simulink model "lane_keeping_fpga_in_the_loop"  (R2025b)
settings: Solver=ode1  StartTime=0.0  StopTime=30.0  RelTol=1e-3
model workspace (MAT data in the model file):
  firstWarning = 1
  originalScenarioChecksum = '9B63FD3C04BCEB1F00254244C35DE55B'
undefined symbols (not defined in the file): gray, Sim3dSensor
libraries: instrumentseriallib x3, simulink_extras x2, visiongeotforms x1, sim3dcameralib x1, sim3dlib x1, sim3dautolib x1
(part 1 of 2)
settings Model: Creator=aless  LastModifiedBy=corne

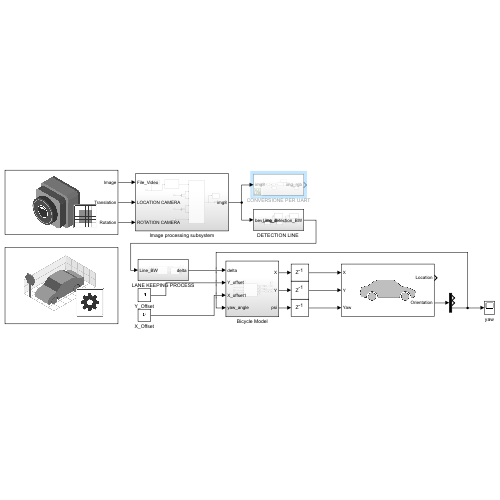
[thumbnail: Simulink's stored preview of the top-level diagram]
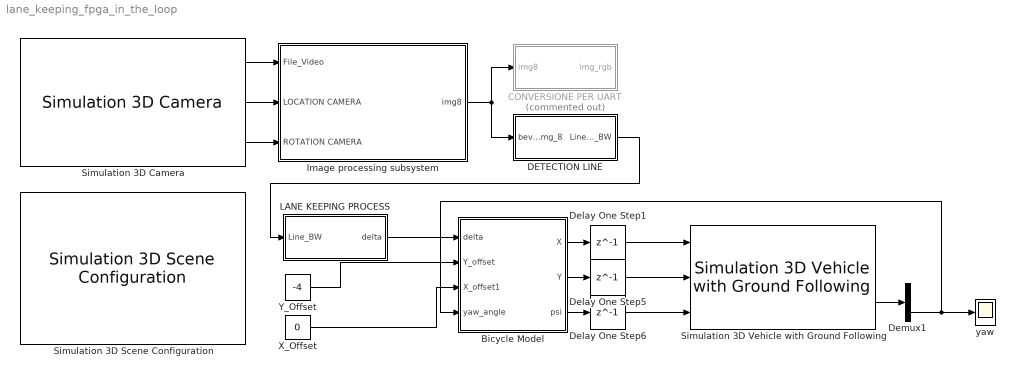
== system lane_keeping_fpga_in_the_loop ==
  Bicycle Model : Subsystem
  CONVERSIONE PER UART : Subsystem  Commented=on
  "DETECTION LINE " : Subsystem
  Delay One Step1 : Delay  DelayLength=1
  Delay One Step5 : Delay  DelayLength=1  InitialCondition=0
  Delay One Step6 : Delay  DelayLength=1
  Demux1 : Demux  Outputs=3
  Image processing subsystem : Subsystem
  LANE KEEPING PROCESS : Subsystem  Description=|
      | -Pulizia immagine
      | -Rotazione bev
      | -Pure pursuit
  Simulation 3D Camera : sim3dcameralib/Simulation 3D Camera  Priority=1  sensorTag=Sim3dSensor�  sensorId=1  sensorName=Sim3dSensor�  vehTagList={'Scene Origin';'ego'}  vehTag=ego  CoordinateSystem=ISO8855  mountLoc=Origin  offsetFlag=on  tmountOffset=[1.2,0,1.6]  extTmount=off  rmountOffset=[0.6,30,21.50]  extRmount=off  FocalLength=[950, 950]  OpticalCenter=[540, 960]  ImageSize=[1080, 1920]  RadialDistortion=[0, 0]  TangentialDistortion=[0, 0]  SensorSkew=0  VisualizeFieldOfView=off  FieldOfViewRange=61  DepthOutportEnabled=off  SemanticOutportEnabled=off  TransformOutportEnabled=on  SampleTime=-1  mountPoint=[1.2 0 1.6]  mountOrientation=[0.6 30 21.5]  aMode=3  ID=1
      settings: LibrarySourceBlock=drivingsim3d/Simulation 3D Camera
  Simulation 3D Scene Configuration : sim3dlib/Simulation 3D Scene Configuration  Priority=0  ProjectFormat=Default Scenes  SceneDesc=Straight road  ProjectName=C:\Program Files\MATLAB\R2025b\toolbox\shared\sim3d_projects\automotive_project_windows\UE\WindowsNoEditor\VehicleSimulation.exe  ScenePath=/Game/Maps/HwStrght  UEProjPath=C:\Users\aless\Desktop\AutoVrtlEnv\AutoVrtlEnv.uproject  EnableOpenDRIVE=off  OpenDRIVEName=C:\Users\aless\Desktop\acav\ACAV PROJECT\asam_prova\prova.xodr  vehTagList={'Custom';'Scene Origin';'ego'}  vehTag=ego  AttachedCameraRelativeTranslation=[0 0 0]  FreeCameraDefaultInitialTranslation=[-6, 0, 2]  AttachedCameraRelativeRotation=[0 0 0]  FreeCameraDefaultInitialRotation=[0, -15, 0]  ViewpointName=Custom  FreeCameraInitialTranslation=[0, 0, 0]  ViewpointTranslation=[0 0 0]  FreeCameraInitialRotation=[0, 0, 0]  ViewpointRotation=[0 0 0]  OpVisEn=off  Ts=1/100  EnableWindow=on  EnableRemoteAccess=off  EnableWeather=off  SunAzimuth=90  SunAltitude=40.0  EnableGeospatialSun=off  Latitude=0  Longitude=0  Date=2023-01-01  Time=10:30:00  GeoTimeZone=-5.0  SunDaylightSaving=off  wind=1  clouds=10  EnableVolumetricClouds=off  CloudCoverage=0  CloudAltitude=6  fog=0  rain=0  RaindropsEffect=off  SnowDensity=0  EnableGeospatial=off  TilesetSource=Earth terrain  UseTrueOrigin=off  OriginHeight=200  OriginLatitude=40.744652  OriginLongitude=-73.988864  MapStyle=Aerial  AdditionalAssetIDs=[]  UseAdvancedSunSky=off  SolarTime=11  TimeZone=-5  Day=21  Month=9  Year=2022  UseDaylightSavingTime=on  DSTStartDay=10  DSTStartMonth=3  DSTEndDay=3  DSTEndMonth=11  DSTSwitchHour=2  sensorTag=MainCamera1  sensorId=1  sensorName=MainCamera1  mountLoc=Origin  offsetFlag=off  tmountOffset=[0, 0, 0]  rmountOffset=[0, 0, 0]  HorizontalResolution=1280  VerticalResolution=720  HorizontalFOV=60  mountPoint=[0 0 0]  mountOrientation=[0 0 0]  aMode=3  ID=1  GeoTrigger=Inactive  ViewNameList={'Custom'}  ViewTranslationList={'[0 0 0]'}  ViewRotationList={'[0 0 0]'}
      settings: LibrarySourceBlock=drivingsim3d/Simulation 3D Scene Configuration
  Simulation 3D Vehicle with Ground Following : sim3dautolib/Simulation 3D Vehicle with Ground Following  Priority=-1  PassVehMesh=Sport utility vehicle  MeshPath=/MathWorksAutomotiveContent/Vehicles/Muscle/Meshes/SK_MuscleCar.SK_MuscleCar  TrackWidth=1.9  WheelBase=3  WheelRadius=0.35  VehColor=Red  CoordinateSystem=ISO8855  InitialPos=[0, -4, 0]  InitialRot=[0, 0, 0]  ActorName=ego  SampleTime=-1  ActorType=SimulinkVehicle  ID=C  aMode=3  ActorTag=ego  CoordinateScheme=0  VehLightsControl=off  HeadlightColor=[ 1, 1, 1 ]  HighBeamIntensity=100000  LowBeamIntensity=60000  HighBeamConeAngle=70  LowBeamConeAngle=70  LeftHeadlightOrientation=[ 0, 0 ]  RightHeadlightOrientation=[ 0, 0 ]  BrakelightIntensity=500  ReverselightIntensity=500  SignallightIntensity=500  SignallightPeriod=1  SignalPulseWidth=50  TransformOutportEnabled=on
      settings: LibrarySourceBlock=drivingsim3d/Simulation 3D Vehicle with Ground Following
  X_Offset : Constant  Value=0
  Y_Offset : Constant  Value=-4
  yaw : Scope
      settings: ActiveDisplayYMinimum=-1.1586010927242787  ActiveDisplayYMaximum=1.3448102951375731  DataLoggingVariableName=ScopeData11
  wires:
  "DETECTION LINE "/1(Line_detection_BW) -> LANE KEEPING PROCESS/1(Line_BW​)
  Image processing subsystem/1(img8) -> CONVERSIONE PER UART/1(img8), "DETECTION LINE "/1(bev_img_8)
  LANE KEEPING PROCESS/1(delta) -> Bicycle Model/1(delta)
  Simulation 3D Camera/1 -> Image processing subsystem/1(File_Video)
  Bicycle Model/2(Y) -> Delay One Step5/1
  Bicycle Model/1(X) -> Delay One Step1/1
  Simulation 3D Vehicle with Ground Following/2 -> Demux1/1
  Simulation 3D Camera/2 -> Image processing subsystem/2(LOCATION CAMERA)
  Simulation 3D Camera/3 -> Image processing subsystem/3(ROTATION CAMERA)
  Delay One Step6/1 -> Simulation 3D Vehicle with Ground Following/3
  Bicycle Model/3(psi) -> Delay One Step6/1
  Demux1/3 -> yaw/1, Bicycle Model/4(yaw_angle)
  Delay One Step1/1 -> Simulation 3D Vehicle with Ground Following/1
  Delay One Step5/1 -> Simulation 3D Vehicle with Ground Following/2
  Y_Offset/1 -> Bicycle Model/2(Y_offset)
  X_Offset/1 -> Bicycle Model/3(X_offset1)

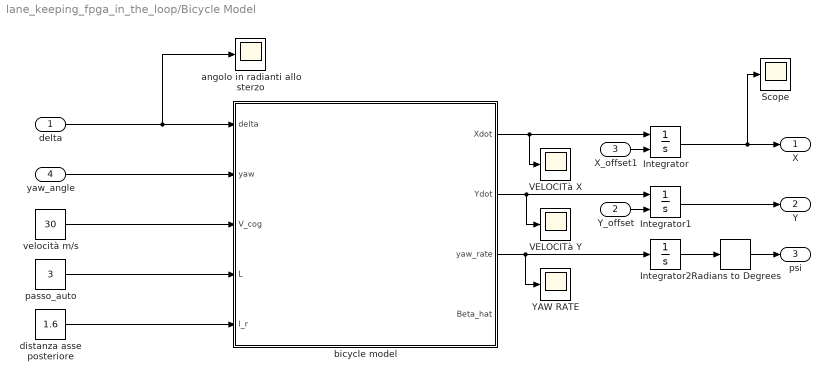
== system lane_keeping_fpga_in_the_loop/Bicycle Model ==
  delta : Inport
  Y_offset : Inport  Port=2
  X_offset1 : Inport  Port=3
  yaw_angle : Inport  Port=4
  Integrator : Integrator  InitialConditionSource=external
  Integrator1 : Integrator  InitialConditionSource=external  InitialCondition=-130
  Integrator2 : Integrator
  Radians to Degrees : simulink_extras/Transformations/Radians to Degrees
  Scope : Scope
      settings: ActiveDisplayYMinimum=-2.3618138795420052  ActiveDisplayYMaximum=7.426328435560519  DataLoggingVariableName=ScopeData5
  VELOCITà X : Scope
      settings: ActiveDisplayYMinimum=-0.055053619065674256  ActiveDisplayYMaximum=1.1172281798961861  DataLoggingVariableName=ScopeData3
  VELOCITà Y : Scope
      settings: ActiveDisplayYMinimum=-1  ActiveDisplayYMaximum=1  DataLoggingVariableName=ScopeData4
  YAW RATE : Scope
      settings: ActiveDisplayYMinimum=-0.13935375186428128  ActiveDisplayYMaximum=0.11342111745280879  DataLoggingVariableName=ScopeData2
  angolo in radianti allo sterzo : Scope
      settings: ActiveDisplayYMinimum=-0.34632467486503338  ActiveDisplayYMaximum=0.4914403733953655
  "bicycle model " : MATLAB Function  TreatAsAtomicUnit=on
  distanza asse posteriore : Constant  Value=1.6
  passo_auto : Constant  Value=3
  "velocità m/s " : Constant  Value=30
  X : Outport
  Y : Outport  Port=2
  psi : Outport  Port=3
  wires:
  "bicycle model "/1(Xdot) -> VELOCITà X/1, Integrator/1
  "bicycle model "/2(Ydot) -> VELOCITà Y/1, Integrator1/1
  Integrator/1 -> X/1, Scope/1
  Integrator1/1 -> Y/1
  delta/1 -> angolo in radianti allo sterzo/1, "bicycle model "/1(delta)
  yaw_angle/1 -> "bicycle model "/2(yaw)
  Radians to Degrees/1 -> psi/1
  "bicycle model "/3(yaw_rate) -> YAW RATE/1, Integrator2/1
  "velocità m/s "/1 -> "bicycle model "/3(V_cog)
  passo_auto/1 -> "bicycle model "/4(L)
  distanza asse posteriore/1 -> "bicycle model "/5(l_r)
  Integrator2/1 -> Radians to Degrees/1
  Y_offset/1 -> Integrator1/2
  X_offset1/1 -> Integrator/2

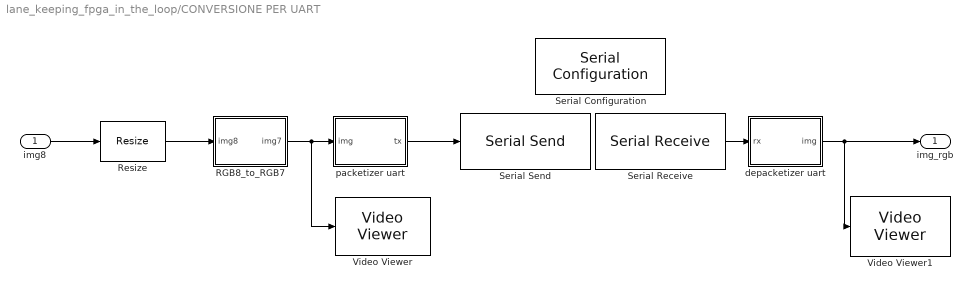
== system lane_keeping_fpga_in_the_loop/CONVERSIONE PER UART ==
  img8 : Inport
  RGB8_to_RGB7 : MATLAB Function  TreatAsAtomicUnit=on
  Resize : visiongeotforms/Resize  specify=Number of output rows and columns  rfactor=[200 150]  outCols=25  outRows=25  outRowsCols=[256 256]  interp_method=Bilinear  antialias=on  useROI=off  roiFlag=off  roundingMode=Nearest  overflowMode=on  prodOutputMode=Binary point scaling  prodOutputWordLength=32  prodOutputFracLength=10
  Serial Configuration : instrumentseriallib/Serial Configuration  Description=il valore del baund rate è uguale a fpga (la massima è 921600 e dipende da usb pc non da fpga)  Priority=-200000  PortSel=COM5  Port=COM5  ComPort=COM5  BaudRate=921600  DataBits=8  Parity=none  StopBits=1  ByteOrder=little-endian  FlowControl=none  Timeout=10  SimulateUsing=Interpreted execution  BlockInModel=on  aMode=1
  Serial Receive : instrumentseriallib/Serial Receive  Priority=1  PortSel=COM5  Port=COM5  ComPort=COM5  DataType=uint8  SaveDataType=uint8  ToggleHeader=on  Header=[255]  ToggleDataSize=on  DataSize=[65536 1]  ToggleTerminator=on  Terminator=Custom terminator  CustomTerminator=[241]  InputFormat=Column major  EnableBlockingMode=on  ActionDataUnavailable=Output last received value  ActionWhenDataUnavailable=Output last received value  CustomValue=0  SampleTime=0.1  SimulateUsing=Interpreted execution  BlockInModel=on  aMode=1  LibraryInUse=instrumentlib
  Serial Send : instrumentseriallib/Serial Send  Priority=1  PortSel=COM5  Port=COM5  ComPort=COM5  Header=[255]  Terminator=Custom terminator  CustomTerminator=[241]  EnableBlockingMode=off  SimulateUsing=Interpreted execution  BlockInModel=on  aMode=1
  Video Viewer : VideoViewer  Description=test di controllo RGB a 7 bit (da 8 bit eseguiamo una divisione per 2 perchè 1 bit degli 8 inviati indica che è l'ultimo bit inviato)  colormapValue=gray(256)  FigPos=[1019 931.666666666667 645 275]
  Video Viewer1 : VideoViewer  colormapValue=gray(256)  FigPos=[878 553.666666666667 845 301]
  depacketizer uart : MATLAB Function  TreatAsAtomicUnit=on
  packetizer uart : MATLAB Function  TreatAsAtomicUnit=on
  img_rgb : Outport
  wires:
  RGB8_to_RGB7/1(img7) -> packetizer uart/1(img), Video Viewer/1
  Serial Receive/1 -> depacketizer uart/1(rx)
  depacketizer uart/1(img) -> Video Viewer1/1, img_rgb/1
  Resize/1 -> RGB8_to_RGB7/1(img8)
  img8/1 -> Resize/1
  packetizer uart/1(tx) -> Serial Send/1

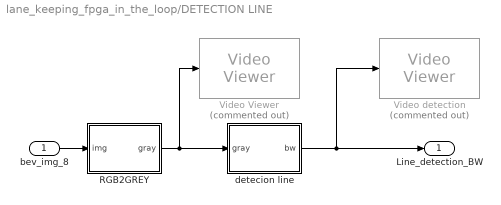
== system lane_keeping_fpga_in_the_loop/DETECTION LINE  ==
  bev_img_8 : Inport
  RGB2GREY : MATLAB Function  TreatAsAtomicUnit=on
  Video Viewer : VideoViewer  Commented=on  colormapValue=gray(256)  FigPos=[1270 462.666666666667 418 304]
  Video detection : VideoViewer  Commented=on  colormapValue=gray(256)  FigPos=[856 1015.66666666667 851 911]
  detecion line : MATLAB Function  TreatAsAtomicUnit=on
  Line_detection_BW : Outport
  wires:
  bev_img_8/1 -> RGB2GREY/1(img)
  RGB2GREY/1(gray) -> Video Viewer/1, detecion line/1(gray)
  detecion line/1(bw) -> Line_detection_BW/1, Video detection/1

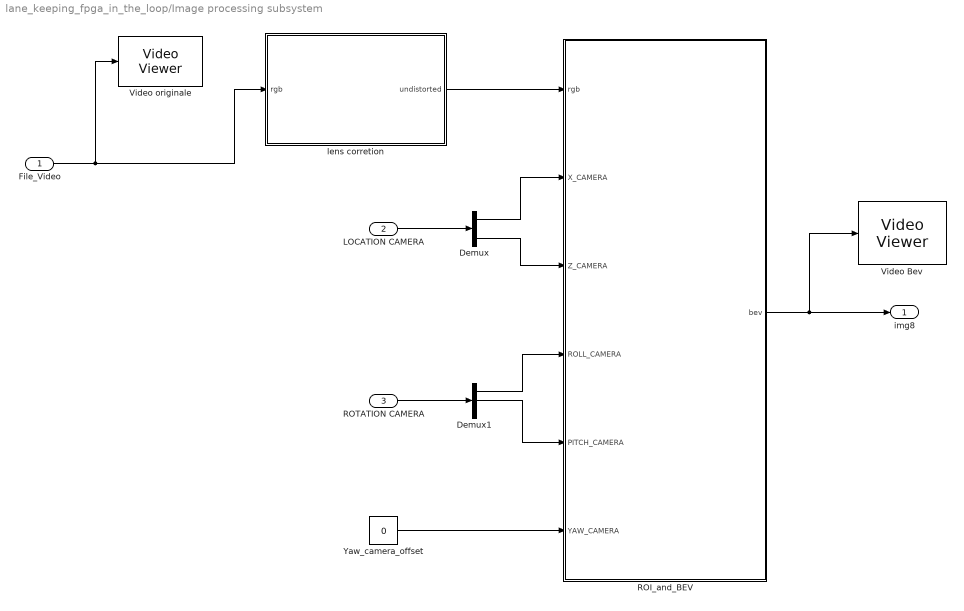
== system lane_keeping_fpga_in_the_loop/Image processing subsystem ==
  File_Video : Inport
  LOCATION CAMERA : Inport  Port=2
  ROTATION CAMERA : Inport  Port=3
  Demux : Demux  Outputs=3
  Demux1 : Demux  Outputs=3
  ROI_and_BEV : MATLAB Function  TreatAsAtomicUnit=on
  Video Bev : VideoViewer  colormapValue=gray(256)  FigPos=[-13 965 1539 768]
  Video originale : VideoViewer  colormapValue=gray(256)  FigPos=[1 814 1536 717]
  Yaw_camera_offset : Constant  Value=0
  lens corretion : MATLAB Function  TreatAsAtomicUnit=on
  img8 : Outport
  wires:
  File_Video/1 -> Video originale/1, lens corretion/1(rgb)
  LOCATION CAMERA/1 -> Demux/1
  lens corretion/1(undistorted) -> ROI_and_BEV/1(rgb)
  ROI_and_BEV/1(bev) -> img8/1, Video Bev/1
  Demux/1 -> ROI_and_BEV/2(X_CAMERA)
  Demux/3 -> ROI_and_BEV/3(Z_CAMERA)
  ROTATION CAMERA/1 -> Demux1/1
  Demux1/1 -> ROI_and_BEV/4(ROLL_CAMERA)
  Demux1/2 -> ROI_and_BEV/5(PITCH_CAMERA)
  Yaw_camera_offset/1 -> ROI_and_BEV/6(YAW_CAMERA)

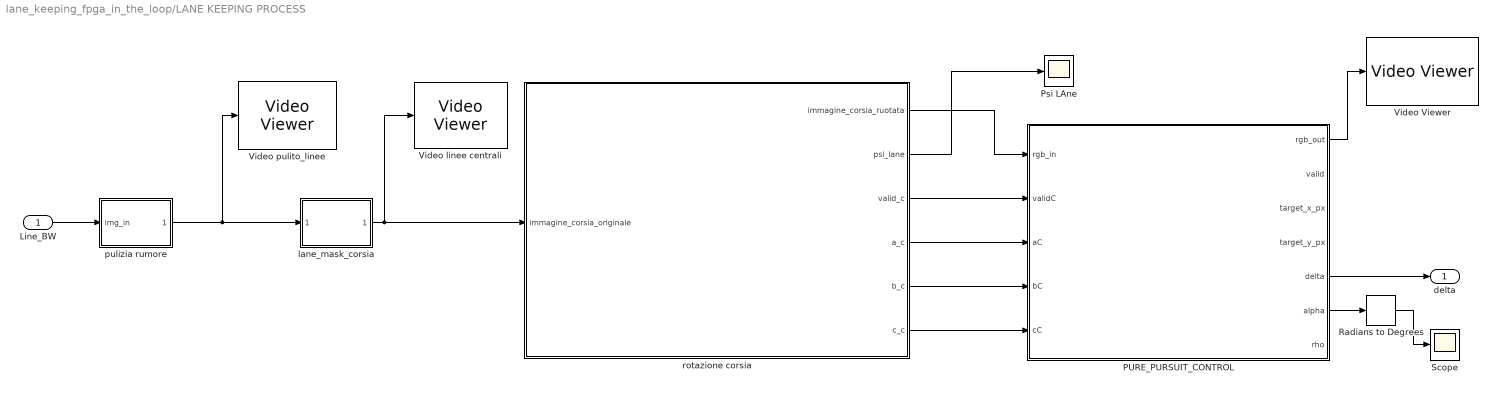
== system lane_keeping_fpga_in_the_loop/LANE KEEPING PROCESS ==
  Line_BW​ : Inport
  PURE_PURSUIT_CONTROL : MATLAB Function  TreatAsAtomicUnit=on
  Psi LAne : Scope
  Radians to Degrees : simulink_extras/Transformations/Radians to Degrees
  Scope : Scope
      settings: ActiveDisplayYMinimum=-21.688585463495443  ActiveDisplayYMaximum=29.571917697196469  DataLoggingVariableName=ScopeData8
  Video Viewer : VideoViewer  colormapValue=gray(256)  FigPos=[1024 631 383 351]
  Video linee centrali : VideoViewer  colormapValue=gray(256)  FigPos=[591 907 851 768]
  Video pulito_linee : VideoViewer  colormapValue=gray(256)  FigPos=[2 1015.66666666667 851 767.66666666667]
  lane_mask_corsia : MATLAB Function  TreatAsAtomicUnit=on
  pulizia rumore : MATLAB Function  TreatAsAtomicUnit=on
  rotazione corsia : Subsystem
  delta : Outport
  wires:
  Line_BW​/1 -> pulizia rumore/1(img_in)
  lane_mask_corsia/1(lane_mask) -> Video linee centrali/1, rotazione corsia/1(immagine_corsia_originale)
  rotazione corsia/1(immagine_corsia_ruotata) -> PURE_PURSUIT_CONTROL/1(rgb_in)
  rotazione corsia/2(psi_lane) -> Psi LAne/1
  rotazione corsia/3(valid_c) -> PURE_PURSUIT_CONTROL/2(validC)
  rotazione corsia/4(a_c) -> PURE_PURSUIT_CONTROL/3(aC)
  rotazione corsia/5(b_c) -> PURE_PURSUIT_CONTROL/4(bC)
  rotazione corsia/6(c_c) -> PURE_PURSUIT_CONTROL/5(cC)
  PURE_PURSUIT_CONTROL/1(rgb_out) -> Video Viewer/1
  Radians to Degrees/1 -> Scope/1
  PURE_PURSUIT_CONTROL/5(delta) -> delta/1
  PURE_PURSUIT_CONTROL/6(alpha) -> Radians to Degrees/1
  pulizia rumore/1(img_out) -> Video pulito_linee/1, lane_mask_corsia/1(binary_img)

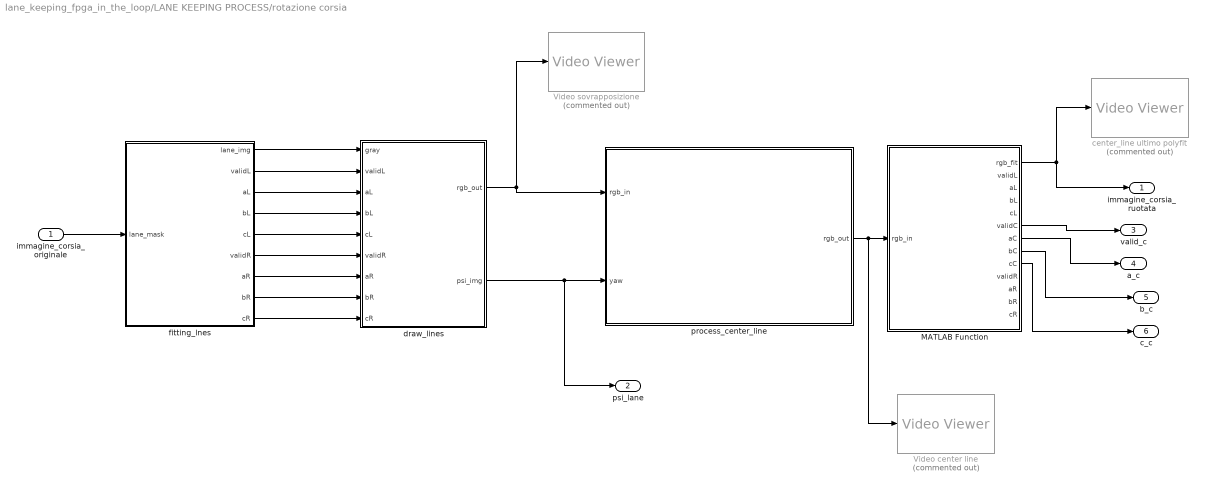
== system lane_keeping_fpga_in_the_loop/LANE KEEPING PROCESS/rotazione corsia ==
  immagine_corsia_originale : Inport
  MATLAB Function : MATLAB Function  TreatAsAtomicUnit=on
  Video center line : VideoViewer  Commented=on  colormapValue=gray(256)  FigPos=[821 1029.66666666667 851 911]
  Video sovrapposizione : VideoViewer  Commented=on  colormapValue=gray(256)  FigPos=[1 1016.66666666667 1707 920]
  center_line ultimo polyfit : VideoViewer  Commented=on  colormapValue=gray(256)  FigPos=[1 1016.66666666667 1707 920]
  draw_lines : MATLAB Function  TreatAsAtomicUnit=on
  fitting_lnes : MATLAB Function  TreatAsAtomicUnit=on
  process_center_line : MATLAB Function  TreatAsAtomicUnit=on
  immagine_corsia_ruotata : Outport
  psi_lane : Outport  Port=2
  valid_c : Outport  Port=3
  a_c : Outport  Port=4
  b_c : Outport  Port=5
  c_c : Outport  Port=6
  wires:
  immagine_corsia_originale/1 -> fitting_lnes/1(lane_mask)
  fitting_lnes/1(lane_img) -> draw_lines/1(gray)
  fitting_lnes/2(validL) -> draw_lines/2(validL)
  fitting_lnes/3(aL) -> draw_lines/3(aL)
  fitting_lnes/4(bL) -> draw_lines/4(bL)
  fitting_lnes/5(cL) -> draw_lines/5(cL)
  fitting_lnes/6(validR) -> draw_lines/6(validR)
  fitting_lnes/7(aR) -> draw_lines/7(aR)
  fitting_lnes/8(bR) -> draw_lines/8(bR)
  fitting_lnes/9(cR) -> draw_lines/9(cR)
  draw_lines/1(rgb_out) -> process_center_line/1(rgb_in), Video sovrapposizione/1
  draw_lines/2(psi_img) -> psi_lane/1, process_center_line/2(yaw)
  process_center_line/1(rgb_out) -> Video center line/1, MATLAB Function/1(rgb_in)
  MATLAB Function/1(rgb_fit) -> center_line ultimo polyfit/1, immagine_corsia_ruotata/1
  MATLAB Function/6(validC) -> valid_c/1
  MATLAB Function/7(aC) -> a_c/1
  MATLAB Function/8(bC) -> b_c/1
  MATLAB Function/9(cC) -> c_c/1

== matlab function lane_keeping_fpga_in_the_loop/LANE KEEPING PROCESS/rotazione corsia/draw_lines ==
  data: gray input; rgb_out output; validL input; aL input; bL input; cL input; validR input; aR input; bR input; cR input; psi_img output double
function [rgb_out, psi_img] = Draw_Lanes_With_Gray(gray, validL, aL, bL, cL, validR, aR, bR, cR)
%#codegen

[H,W] = size(gray);

rgb_out = zeros(H,W,3,'uint8');
psi_img = 0.0;
%curve_gray = zeros(H,W,'uint8');
%center_gray = zeros(H,W,'uint8');

for r = 1:H
    for c = 1:W
        val = gray(r,c);
        rgb_out(r,c,1) = val;
        rgb_out(r,c,2) = val;
        rgb_out(r,c,3) = val;
    end
end

thickness_lane   = int32(1);
thickness_center = int32(1);

for r = 1:H

    y = double(r);

    %xL = 0.0;
    %xR = 0.0;

    % =====================================================
    % Linea sinistra
    % =====================================================
    if validL
        xL = aL*y*y + bL*y + cL;
        colL = int32(round(xL));

        for dc = -thickness_lane:thickness_lane
            cc = colL + dc;

            if cc >= 1 && cc <= W
                % corsia bianca
                rgb_out(r,cc,1) = uint8(255);
                rgb_out(r,cc,2) = uint8(255);
                rgb_out(r,cc,3) = uint8(255);

                %curve_gray(r,cc) = uint8(255);
            end
        end
    end

    % =====================================================
    % Linea destra
    % =====================================================
    if validR
        xR = aR*y*y + bR*y + cR;
        colR = int32(round(xR));

        for dc = -thickness_lane:thickness_lane
            cc = colR + dc;

            if cc >= 1 && cc <= W
                % corsia bianca
                rgb_out(r,cc,1) = uint8(255);
                rgb_out(r,cc,2) = uint8(255);
                rgb_out(r,cc,3) = uint8(255);

                %curve_gray(r,cc) = uint8(255);
            end
        end
    end

       % =====================================================
        % Centerline blu
        % =====================================================
        if validL && validR
        
            % coefficienti centerline
        aC = 0.5*(aL + aR);
        bC = 0.5*(bL + bR);
        cC = 0.5*(cL + cR);
        
        % riga più bassa
        y0 = double(H);
        
        % derivata dx/dy alla base
        mC0 = 2.0*aC*y0 + bC;
        
        % angolo rispetto alla verticale immagine [rad]
        psi_img = atan(mC0);
        
        xC = aC*y*y + bC*y + cC;
        colC = int32(round(xC));
    
        for dc = -thickness_center:thickness_center
            cc = colC + dc;
    
            if cc >= 1 && cc <= W
                rgb_out(r,cc,1) = uint8(0);
                rgb_out(r,cc,2) = uint8(0);
                rgb_out(r,cc,3) = uint8(255);
    
                %center_gray(r,cc) = uint8(255);
            end
        end
    end

end

end

== matlab function lane_keeping_fpga_in_the_loop/LANE KEEPING PROCESS/rotazione corsia/process_center_line ==
  data: rgb_in input; rgb_out output uint8 size=[256 256 3]; yaw input
function rgb_out = Rotate_Image_Yaw_2D(rgb_in, yaw)
%#codegen
%
% yaw [rad]
% positivo = rotazione antioraria nell'immagine

[H,W,~] = size(rgb_in);

rgb_out = zeros(H,W,3,'uint8');

cx = double(W)/2.0;
cy = double(H)/2.0;

c = cos(yaw);
s = sin(yaw);

% =========================================================
% Inverse mapping:
% per ogni pixel output trovo da dove leggere nell'input
% =========================================================
for r_out = 1:H
    for c_out = 1:W

        x_out = double(c_out) - cx;
        y_out = double(r_out) - cy;

        % rotazione inversa: -yaw
        x_in =  c*x_out + s*y_out;
        y_in = -s*x_out + c*y_out;

        c_in = int32(round(x_in + cx));
        r_in = int32(round(y_in + cy));

        if r_in >= 1 && r_in <= H && c_in >= 1 && c_in <= W
            rgb_out(r_out,c_out,1) = rgb_in(r_in,c_in,1);
            rgb_out(r_out,c_out,2) = rgb_in(r_in,c_in,2);
            rgb_out(r_out,c_out,3) = rgb_in(r_in,c_in,3);
        end
    end
end

end

== matlab function lane_keeping_fpga_in_the_loop/LANE KEEPING PROCESS/rotazione corsia/MATLAB Function ==
  data: rgb_in input; rgb_fit output; validL output; aL output; bL output; cL output; validC output; aC output; bC output; cC output; validR output; aR output; bR output; cR output
function [rgb_fit, validL, aL, bL, cL, validC, aC, bC, cC, validR, aR, bR, cR] = Fit_Lanes_From_Blue_Center(rgb_in)
%#codegen
%
% Modello:
%   x(y) = a*y^2 + b*y + c

[H,W,~] = size(rgb_in);

rgb_fit = zeros(H,W,3,'uint8');

validL = false; validC = false; validR = false;
aL = 0.0; bL = 0.0; cL = 0.0;
aC = 0.0; bC = 0.0; cC = 0.0;
aR = 0.0; bR = 0.0; cR = 0.0;

min_points = int32(20);
thickness = int32(1);

% copia input
for r = 1:H
    for c = 1:W
        rgb_fit(r,c,1) = rgb_in(r,c,1);
        rgb_fit(r,c,2) = rgb_in(r,c,2);
        rgb_fit(r,c,3) = rgb_in(r,c,3);
    end
end

% =========================================================
% 1) Fit centerline dai punti blu
% =========================================================
S0C = 0.0; S1C = 0.0; S2C = 0.0; S3C = 0.0; S4C = 0.0;
T0C = 0.0; T1C = 0.0; T2C = 0.0;
nC = int32(0);

for r = 1:H
    y = double(r);
    y2 = y*y;
    y3 = y2*y;
    y4 = y2*y2;

    for c = 1:W
        Rv = rgb_in(r,c,1);
        Gv = rgb_in(r,c,2);
        Bv = rgb_in(r,c,3);

        is_blue = Rv < 80 && Gv < 80 && Bv > 150;

        if is_blue
            x = double(c);

            S0C = S0C + 1.0;
            S1C = S1C + y;
            S2C = S2C + y2;
            S3C = S3C + y3;
            S4C = S4C + y4;

            T0C = T0C + x;
            T1C = T1C + y*x;
            T2C = T2C + y2*x;

            nC = nC + 1;
        end
    end
end

if nC < min_points
    return;
end

[okC, aC_tmp, bC_tmp, cC_tmp] = solve_quad_fit(S0C,S1C,S2C,S3C,S4C,T0C,T1C,T2C);

if ~okC
    return;
end

validC = true;
aC = aC_tmp;
bC = bC_tmp;
cC = cC_tmp;

% =========================================================
% 2) Usando la centerline, cerco i primi bianchi SX/DX
% =========================================================
S0L = 0.0; S1L = 0.0; S2L = 0.0; S3L = 0.0; S4L = 0.0;
T0L = 0.0; T1L = 0.0; T2L = 0.0;
nL = int32(0);

S0R = 0.0; S1R = 0.0; S2R = 0.0; S3R = 0.0; S4R = 0.0;
T0R = 0.0; T1R = 0.0; T2R = 0.0;
nR = int32(0);

for r = 1:H

    y = double(r);
    y2 = y*y;
    y3 = y2*y;
    y4 = y2*y2;

    xC = aC*y*y + bC*y + cC;
    colC = int32(round(xC));

    if colC < 1
        colC = int32(1);
    end
    if colC > W
        colC = int32(W);
    end

    % -------------------------
    % primo bianco a sinistra
    % -------------------------
    foundL = false;
    xL = int32(0);

    for c = colC:-1:1
        Rv = rgb_in(r,c,1);
        Gv = rgb_in(r,c,2);
        Bv = rgb_in(r,c,3);

        is_white = Rv > 200 && Gv > 200 && Bv > 200;

        if ~foundL && is_white
            xL = int32(c);
            foundL = true;
        end
    end

    if foundL
        x = double(xL);

        S0L = S0L + 1.0;
        S1L = S1L + y;
        S2L = S2L + y2;
        S3L = S3L + y3;
        S4L = S4L + y4;

        T0L = T0L + x;
        T1L = T1L + y*x;
        T2L = T2L + y2*x;

        nL = nL + 1;
    end

    % -------------------------
    % primo bianco a destra
    % -------------------------
    foundR = false;
    xR = int32(0);

    for c = colC:W
        Rv = rgb_in(r,c,1);
        Gv = rgb_in(r,c,2);
        Bv = rgb_in(r,c,3);

        is_white = Rv > 200 && Gv > 200 && Bv > 200;

        if ~foundR && is_white
            xR = int32(c);
            foundR = true;
        end
    end

    if foundR
        x = double(xR);

        S0R = S0R + 1.0;
        S1R = S1R + y;
        S2R = S2R + y2;
        S3R = S3R + y3;
        S4R = S4R + y4;

        T0R = T0R + x;
        T1R = T1R + y*x;
        T2R = T2R + y2*x;

        nR = nR + 1;
    end
end

% =========================================================
% 3) Fit sinistra e destra
% =========================================================
if nL >= min_points
    [okL, aa, bb, cc] = solve_quad_fit(S0L,S1L,S2L,S3L,S4L,T0L,T1L,T2L);
    if okL
        validL = true;
        aL = aa; bL = bb; cL = cc;
    end
end

if nR >= min_points
    [okR, aa, bb, cc] = solve_quad_fit(S0R,S1R,S2R,S3R,S4R,T0R,T1R,T2R);
    if okR
        validR = true;
        aR = aa; bR = bb; cR = cc;
    end
end

% =========================================================
% 4) Disegno fit finale
% =========================================================
rgb_fit(:,:,:) = uint8(0);

for r = 1:H
    y = double(r);

    if validL
        x = aL*y*y + bL*y + cL;
        col = int32(round(x));
        for dc = -thickness:thickness
            cc = col + dc;
            if cc >= 1 && cc <= W
                rgb_fit(r,cc,1) = uint8(255);
                rgb_fit(r,cc,2) = uint8(255);
                rgb_fit(r,cc,3) = uint8(255);
            end
        end
    end

    if validC
        x = aC*y*y + bC*y + cC;
        col = int32(round(x));
        for dc = -thickness:thickness
            cc = col + dc;
            if cc >= 1 && cc <= W
                rgb_fit(r,cc,1) = uint8(0);
                rgb_fit(r,cc,2) = uint8(0);
                rgb_fit(r,cc,3) = uint8(255);
            end
        end
    end

    if validR
        x = aR*y*y + bR*y + cR;
        col = int32(round(x));
        for dc = -thickness:thickness
            cc = col + dc;
            if cc >= 1 && cc <= W
                rgb_fit(r,cc,1) = uint8(255);
                rgb_fit(r,cc,2) = uint8(255);
                rgb_fit(r,cc,3) = uint8(255);
            end
        end
    end
end

end


function [ok, a, b, c] = solve_quad_fit(S0,S1,S2,S3,S4,T0,T1,T2)
%#codegen

ok = false;
a = 0.0; b = 0.0; c = 0.0;

A11 = S4; A12 = S3; A13 = S2;
A21 = S3; A22 = S2; A23 = S1;
A31 = S2; A32 = S1; A33 = S0;

B1 = T2;
B2 = T1;
B3 = T0;

detA = A11*(A22*A33 - A23*A32) ...
     - A12*(A21*A33 - A23*A31) ...
     + A13*(A21*A32 - A22*A31);

if abs(detA) < 1e-9
    return;
end

detA_a = B1*(A22*A33 - A23*A32) ...
       - A12*(B2*A33 - A23*B3) ...
       + A13*(B2*A32 - A22*B3);

detA_b = A11*(B2*A33 - A23*B3) ...
       - B1*(A21*A33 - A23*A31) ...
       + A13*(A21*B3 - B2*A31);

detA_c = A11*(A22*B3 - B2*A32) ...
       - A12*(A21*B3 - B2*A31) ...
       + B1*(A21*A32 - A22*A31);

a = detA_a / detA;
b = detA_b / detA;
c = detA_c / detA;

ok = true;

end

== matlab function lane_keeping_fpga_in_the_loop/LANE KEEPING PROCESS/PURE_PURSUIT_CONTROL ==
  data: rgb_in input; rgb_out output; validC input; aC input; bC input; cC input; valid output; target_x_px output; target_y_px output; delta output; alpha output; rho output
function [rgb_out, valid, target_x_px, target_y_px, delta, alpha, rho] = PurePursuit_From_Fitted_Center(rgb_in, validC, aC, bC, cC)
%#codegen
%
% =========================================================
% PURE PURSUIT CONTROL FROM FITTED BLUE CENTERLINE
% =========================================================
%
% Input:
%   rgb_in  : immagine RGB 256x256, tipicamente rgb_fit
%   validC  : true se la centerline è valida
%   aC,bC,cC: coefficienti della centerline:
%
%               x(y) = aC*y^2 + bC*y + cC
%
% Output:
%   rgb_out      : immagine debug
%   valid        : true se il target lookahead è valido
%   target_x_px  : colonna target [px]
%   target_y_px  : riga target [px]
%   delta        : angolo sterzo [rad]
%   alpha        : angolo del lookahead point [rad]
%   rho        : curvatura Pure Pursuit [1/m]
%
% Convenzioni:
%   X positivo avanti
%   Y positivo sinistra
%   delta > 0 sterza a sinistra
%
% Immagine:
%   riga cresce verso il basso
%   colonna cresce verso destra

[H,W,~] = size(rgb_in);

% =========================================================
% Output iniziali
% =========================================================
rgb_out = rgb_in;

valid = false;

target_x_px = int32(round(double(W)/2.0));
target_y_px = int32(H);

delta = 0.0;
alpha = 0.0;
rho = 0.0;

if ~validC
    return;
end

% =========================================================
% Parametri veicolo / immagine
% =========================================================
L = 3;                 % [m] passo veicolo
delta_max = 1;        % [rad] circa 30 deg

pixels_per_meter_x = 25.6;   % [px/m] scala laterale
pixels_per_meter_y = 25.6;   % [px/m] scala longitudinale (BEV 10MX10M = 256pxX256px)

d_la = 5.0;           % [m] distanza lookahead desiderata

% Posizione ego in pixel
ego_x_px = double(W)/2.0;
ego_y_px = double(H);

% =========================================================
% 1) Cerca sulla parabola il punto più vicino a d_la
% =========================================================
%
% Modello immagine:
%   xC(r) = aC*r^2 + bC*r + cC
%
% Conversione metrica:
%   X = (ego_y_px - r)/pixels_per_meter_y
%   Y = -(xC - ego_x_px)/pixels_per_meter_x
%
% Distanza:
%   d = sqrt(X^2 + Y^2)
%
% Cerchiamo il punto della centerline con:
%   d ~= d_la
%

best_err = 1.0e9;
best_r = int32(H);
best_c = int32(round(ego_x_px));

found = false;

for r = 1:H

    y = double(r);

    xC = aC*y*y + bC*y + cC;
    c_px = int32(round(xC));

    if c_px >= 1 && c_px <= W

        X_m = (ego_y_px - y) / pixels_per_meter_y;
        Y_m = -(xC - ego_x_px) / pixels_per_meter_x;

        % Consideriamo solo punti davanti al veicolo
        if X_m > 0.05

            d_m = sqrt(X_m*X_m + Y_m*Y_m);
            err = abs(d_m - d_la);

            if err < best_err
                best_err = err;
                best_r = int32(r);
                best_c = c_px;
                found = true;
            end
        end
    end
end

if ~found
    return;
end

target_x_px = best_c;
target_y_px = best_r;

% =========================================================
% 2) Coordinate metriche del lookahead point
% =========================================================
r_la = double(target_y_px);
c_la = double(target_x_px);

X_la = (ego_y_px - r_la) / pixels_per_meter_y;      % [m]
Y_la = -(c_la - ego_x_px) / pixels_per_meter_x;     % [m]

d_la = sqrt(X_la*X_la + Y_la*Y_la);

if d_la < 0.1
    return;
end

% =========================================================
% 3) Pure Pursuit
% =========================================================
%
% Angolo del punto lookahead:
%
%   alpha = atan2(Y_la, X_la)
%
% Curvatura arco: (1/raggio)
%
%   rho = 2*sin(alpha)/d_la
%
% Poiché:
%
%   sin(alpha) = Y_la/d_la
%
% allora equivalentemente:
%
%   rho = 2*Y_la/d_la^2
%
% Sterzo cinematic bicycle:
%
%   delta = atan(L*rho)
%

alpha = atan2(Y_la, X_la);

rho = 2.0 * sin(alpha) / d_la;

delta = atan(L * rho);

% Saturazione sterzo
if delta > delta_max
    delta = delta_max;
end

if delta < -delta_max
    delta = -delta_max;
end

valid = true;

% =========================================================
% 4) Debug grafico
% =========================================================

% Disegno centerline verde
for r = 1:H

    y = double(r);
    xC = aC*y*y + bC*y + cC;
    c_px = int32(round(xC));

    if c_px >= 1 && c_px <= W
        rgb_out(r,c_px,1) = uint8(0);
        rgb_out(r,c_px,2) = uint8(255);
        rgb_out(r,c_px,3) = uint8(0);
    end
end

% Disegno ego in rosso
ego_c_i = int32(round(ego_x_px));
ego_r_i = int32(round(ego_y_px));

for dr = -2:2
    for dc = -2:2
        rr = ego_r_i + dr;
        cc = ego_c_i + dc;

        if rr >= 1 && rr <= H && cc >= 1 && cc <= W
            rgb_out(rr,cc,1) = uint8(255);
            rgb_out(rr,cc,2) = uint8(0);
            rgb_out(rr,cc,3) = uint8(0);
        end
    end
end

% Disegno target lookahead in giallo
for dr = -3:3
    for dc = -3:3
        rr = target_y_px + dr;
        cc = target_x_px + dc;

        if rr >= 1 && rr <= H && cc >= 1 && cc <= W
            rgb_out(rr,cc,1) = uint8(255);
            rgb_out(rr,cc,2) = uint8(255);
            rgb_out(rr,cc,3) = uint8(0);
        end
    end
end

% Disegno segmento ego-target in magenta, discretizzato semplice
Nline = int32(60);

for i = 0:Nline

    lambda = double(i) / double(Nline);

    cc_f = ego_x_px + lambda*(double(target_x_px) - ego_x_px);
    rr_f = ego_y_px + lambda*(double(target_y_px) - ego_y_px);

    cc = int32(round(cc_f));
    rr = int32(round(rr_f));

    if rr >= 1 && rr <= H && cc >= 1 && cc <= W
        rgb_out(rr,cc,1) = uint8(255);
        rgb_out(rr,cc,2) = uint8(0);
        rgb_out(rr,cc,3) = uint8(255);
    end
end

end

== matlab function lane_keeping_fpga_in_the_loop/Bicycle Model/bicycle model  ==
  data: delta input; Xdot output; yaw input; V_cog input; L input; l_r input; Ydot output; yaw_rate output; Beta_hat output
function [Xdot,Ydot,yaw_rate, Beta_hat]= fcn(delta,yaw, V_cog, L, l_r)


Beta_hat = atan(l_r/L*tan(delta));

Xdot = V_cog*cos(yaw+Beta_hat);
Ydot = V_cog*sin(yaw+Beta_hat);

yaw_rate = V_cog/L*tan(delta)*cos(Beta_hat);

== matlab function lane_keeping_fpga_in_the_loop/CONVERSIONE PER UART/RGB8_to_RGB7 ==
  data: img8 input; img7 output
function img7 = RGB8_to_RGB7(img8)
%#codegen
img7 = bitshift(img8, -1);
end

== matlab function lane_keeping_fpga_in_the_loop/CONVERSIONE PER UART/packetizer uart ==
  data: img input; tx output
function tx = Pack_UART_Payload(img)
%#codegen
% img: 256x256x3 uint8
% tx : 65536*3x1 uint8

H = 256;
W = 256;

tx = zeros(65536*3,1,'uint8');

k = 1;

for i = 1:H
    for j = 1:W
        tx(k) = img(i,j,1); k = k + 1;
        tx(k) = img(i,j,2); k = k + 1;
        tx(k) = img(i,j,3); k = k + 1;
    end
end

== matlab function lane_keeping_fpga_in_the_loop/CONVERSIONE PER UART/depacketizer uart ==
  data: rx input; img output
function img = Unpack_UART_Payload(rx)
%#codegen
% rx  : 65536x1 uint8
% img : 256x256 uint8

H = 256;
W = 256;

img = zeros(H, W, 'uint8');

k = 1;
for i = 1:H
    for j = 1:W
        img(i,j) = 2*rx(k);%usiamo 2* per fare shift e dare 8 bit al colore
        k = k + 1;
    end
end
end

== matlab function lane_keeping_fpga_in_the_loop/DETECTION LINE /RGB2GREY ==
  data: img input; gray output
function gray = RGB_to_GRAY(img)
%#codegen
% img  : 256x256x3 uint8
% gray : 256x256 uint8
%
% g = (R + G + B)/3

R = uint16(img(:,:,1));
G = uint16(img(:,:,2));
B = uint16(img(:,:,3));

gray16 = floor((R + G + B) / 3);
gray = uint8(gray16);
end

== matlab function lane_keeping_fpga_in_the_loop/DETECTION LINE /detecion line ==
  data: gray input; bw output
function bw = LineDetectionConv(gray)
%#codegen
% gray: 128x128 uint8
% bw  : 128x128 uint8 binaria

bw = zeros(256,256,'uint8');

% Kernel Laplaciano 8-neighbors
K = int16([ 1  1  1;
            1 -8  1;
            1  1  1]);

th = int16(190);   % soglia iniziale da tarare

for i = 2:255
    for j = 2:255
        conv_val = int16(0);

        conv_val = conv_val + int16(gray(i-1,j-1)) * K(1,1);
        conv_val = conv_val + int16(gray(i-1,j  )) * K(1,2);
        conv_val = conv_val + int16(gray(i-1,j+1)) * K(1,3);

        conv_val = conv_val + int16(gray(i  ,j-1)) * K(2,1);
        conv_val = conv_val + int16(gray(i  ,j  )) * K(2,2);
        conv_val = conv_val + int16(gray(i  ,j+1)) * K(2,3);

        conv_val = conv_val + int16(gray(i+1,j-1)) * K(3,1);
        conv_val = conv_val + int16(gray(i+1,j  )) * K(3,2);
        conv_val = conv_val + int16(gray(i+1,j+1)) * K(3,3);

        % valore assoluto
        if conv_val < 0
            conv_val = -conv_val;
        end

        % threshold
        if conv_val >= th
            bw(i,j) = uint8(255);
        else
            bw(i,j) = uint8(0);
        end
    end
end
end

== matlab function lane_keeping_fpga_in_the_loop/LANE KEEPING PROCESS/pulizia rumore ==
  data: img_in input; img_out output
function img_out = Remove_Isolated_White_Pixels(img_in)
% Mantiene validi solo i pixel bianchi che hanno almeno
% un pixel bianco adiacente negli 8 vicini.
%
% Input:
%   img_in  = immagine grayscale oppure binaria
%
% Output:
%   img_out = immagine filtrata

% Dimensioni immagine
[H, W] = size(img_in);

% Output inizializzato nero
img_out = zeros(H, W, 'like', img_in);

% Soglia per decidere se un pixel è bianco
threshold = 128;

% Scorro tutti i pixel interni
for r = 3:H-2
    for c = 3:W-2
        
        % Pixel centrale bianco?
        if img_in(r,c) > threshold
            
            % Controllo i 24 vicini
            hasNeighbor = false;
            
            for dr = -2:2
                for dc = -2:2
                    
                    % Salto il pixel centrale
                    if ~(dr == 0 && dc == 0)
                        if img_in(r+dr, c+dc) > threshold
                            hasNeighbor = true;
                        end
                    end
                    
                end
            end
            
            % Se ha almeno un vicino bianco, lo mantengo
            if hasNeighbor
                img_out(r,c) = img_in(r,c);
            end
            
        end
    end
end

end

== matlab function lane_keeping_fpga_in_the_loop/Image processing subsystem/lens corretion ==
  data: rgb input; undistorted output
    function undistorted = Camera_LensCorrection(rgb)
%#codegen
% Correzione distorsione lente su frame RGB
%
% Input:
%   rgb : frame RGB uint8 HxWx3
%   fx, fy : focali [px]
%   cx, cy : centro ottico [px]
%   k1,k2,k3 : distorsione radiale
%   t1,t2 : distorsione tangenziale

fx = 950;
fy = 950;
cx = 540;
cy = 960;
k1 = 0;
k2 = 0;
k3 = 0;
p1 = 0;
p2 = 0;
%
% Output:
%   undistorted : frame RGB corretto

[H,W,~] = size(rgb);

undistorted = zeros(H,W,3,'uint8');

for v_out = 1:H
    for u_out = 1:W

        % =====================================================
        % 1) Coordinate pixel corrette -> coordinate normalizzate
        % =====================================================
        x = (double(u_out) - cx) / fx;
        y = (double(v_out) - cy) / fy;

        % =====================================================
        % 2) Modello di distorsione
        %    Da pixel ideale/corretto -> pixel distorto
        % =====================================================
        r2 = x*x + y*y;
        r4 = r2*r2;
        r6 = r4*r2;

        radial = 1 + k1*r2 + k2*r4 + k3*r6;

        x_dist = x*radial + 2*p1*x*y + p2*(r2 + 2*x*x);
        y_dist = y*radial + p1*(r2 + 2*y*y) + 2*p2*x*y;

        % =====================================================
        % 3) Coordinate normalizzate distorte -> pixel input
        % =====================================================
        u_in = fx*x_dist + cx;
        v_in = fy*y_dist + cy;

        ui = int32(round(u_in));
        vi = int32(round(v_in));

        % =====================================================
        % 4) Campionamento immagine originale
        % =====================================================
        if ui >= 1 && ui <= W && vi >= 1 && vi <= H
            undistorted(v_out,u_out,1) = rgb(vi,ui,1);
            undistorted(v_out,u_out,2) = rgb(vi,ui,2);
            undistorted(v_out,u_out,3) = rgb(vi,ui,3);
        end
    end
end

end

== matlab function lane_keeping_fpga_in_the_loop/Image processing subsystem/ROI_and_BEV ==
  data: rgb input; bev output; X_CAMERA input; Z_CAMERA input; ROLL_CAMERA input; PITCH_CAMERA input; YAW_CAMERA input
function bev = BEV_From_RGB(rgb, X_CAMERA, Z_CAMERA, ROLL_CAMERA, PITCH_CAMERA, YAW_CAMERA)
%#codegen
% Input : rgb [1080 x 1920 x 3] uint8
% Output: bev [256 x 256 x 3] uint8
%avanti veicolo X  -> profondità camera Zc
%sinistra veicolo Y -> -Xc
%alto veicolo Z     -> -Yc
% ROLL PITCH E YAW CAMERA è GIà IN RADIANTI

A = [ 0  1  0;
      0  0 -1;
      1  0  0 ];

% =========================================================
% 1) Dimensioni immagine originale
% =========================================================
Himg = 1080;
Wimg = 1920;

% =========================================================
% 2) Dimensioni BEV
% =========================================================
Hbev = 256;
Wbev = 256;

bev = zeros(Hbev, Wbev, 3, 'uint8');

% =========================================================
% 3) Intrinseci camera
% =========================================================
fx = 950;
fy = 950;
cx = 960;
cy = 540;

K = [fx  0 cx 0;
      0 fy cy 0;
      0  0  1 0];

% =========================================================
% 4) Posizione camera rispetto al veicolo/mondo
% =========================================================
C = [1.2;
     0;
     1.6];

% =========================================================
% 5) Rotazioni camera [Roll Pitch Yaw] in gradi
% =========================================================
roll  = 0 * pi/180;
pitch = 7.875 * pi/180;
yaw   = -0.4 * pi/180 + YAW_CAMERA; %è l'angolo di imbardata che deve raddrizzare il bev

cr = cos(roll);  sr = sin(roll);
cp = cos(pitch); sp = sin(pitch);
cyaw = cos(yaw); syaw = sin(yaw);

Rx = [1  0   0;
      0  cr sr;
      0  -sr  cr];

Ry = [ cp 0 -sp;
       0  1 0;
      sp 0 cp];

Rz = [cyaw syaw 0;
      -syaw  cyaw 0;
      0     0    1];

% Convenzione usata:YAW-ROLL-PITCH
R_vehicle = Ry * Rx * Rz;

%rotazione assi telecamera = world
R = A*R_vehicle;

% Traslazione mondo -> camera
t = -R * C;

% Matrice di proiezione
P = K * [R t;
        0 0 0 1];

% =========================================================
% 6) Area reale rappresentata nella BEV
% =========================================================
% X = direzione avanti [m]
% Y = direzione laterale [m]
Xmin = 5 ;
Xmax = 15;

Ymin = -5 ;
Ymax = 5 ;

% =========================================================
% 7) Inverse mapping: BEV -> mondo -> immagine
% =========================================================
for rb = 1:Hbev

    % rb = 1 parte lontana, rb = Hbev parte vicina
    Xw = Xmax - (rb-1) * (Xmax - Xmin) / (Hbev-1);
    
    for cb = 1:Wbev

        Yw = Ymin + (cb-1) * (Ymax - Ymin) / (Wbev-1);
        

        % Piano strada
        Zw = 0.0;

        Ow = [Xw; Yw; Zw; 1.0];

        q = P * Ow;

        s = q(3);%zc

        if s > 0

            u = q(1) / s;%xc/zc
            v = q(2) / s;%yc/zc
        
            ui = int32(round(u));
            vi = int32(round(v));
        
            if ui >= 1 && ui <= Wimg && vi >= 1 && vi <= Himg
                bev(rb, cb, 1) = rgb(vi, ui, 1);
                bev(rb, cb, 2) = rgb(vi, ui, 2);
                bev(rb, cb, 3) = rgb(vi, ui, 3);
            else
                % Davanti alla camera ma fuori immagine
                bev(rb, cb, 1) = 255;   % rosso
                bev(rb, cb, 2) = 0;
                bev(rb, cb, 3) = 0;
            end
        
        else
            % Dietro la camera oppure profondità negativa/nulla
            bev(rb, cb, 1) = 0;
            bev(rb, cb, 2) = 0;
            bev(rb, cb, 3) = 255;       % blu
        end
    end
end
